simulink model "PolePlacement_Complete_2019"  (R2019a)
settings: Solver=VariableStepAuto  StartTime=0.0  StopTime=10.0  RelTol=1e-3
values from neighbouring files (symbols this model uses):
  k = place(A, B, new_pole)    [PolePlacement_Controller_script.m]
  K_eta = K_en(5)    [PolePlacement_Controller_script.m]
  K_x = K_en(1:4)    [PolePlacement_Controller_script.m]
  Kr = 1/Kdc(1)    [PolePlacement_Controller_script.m]
  L = C_comp*TF(1)    [LQR_Controller.m]    (also in PolePlacement_Controller_script.m = place(sysestc.A',sysestc.C', 10*new_pole)')
  sysestc = d2c(sysest)    [Controller.m]    (also in LQR_Controller.m; PolePlacement_Controller_script.m)
undefined symbols (not defined in the file or in its folder): sigbuilder_block, v_a_max
libraries: simulink_extras x2
settings Model: Creator=jesuc  LastModifiedBy=arco
settings DebuggingCC: SFMachineParentedDataDiag=error

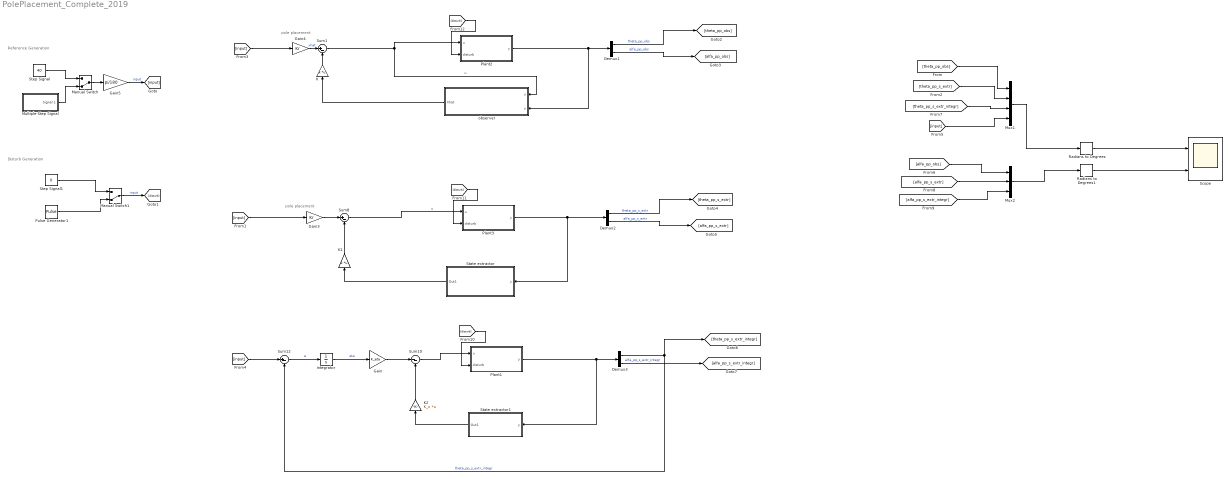
== system PolePlacement_Complete_2019 ==
  note: pole placement
  note: Reference Generation
  note: Disturb Generation
  note: pole placement
  Demux1 : Demux  Outputs=2
  Demux2 : Demux  Outputs=2
  Demux3 : Demux  Outputs=2
  Gain : Gain  Gain=K_eta
  Gain3 : Gain  Gain=Kr
  Gain4 : Gain  Gain=Kr
  Gain5 : Gain  Gain=pi/180
  Integrator : Integrator
  K : Gain  Gain=k  Multiplication=Matrix(K*u)
  K1 : Gain  Gain=k  Multiplication=Matrix(K*u)
  K2 : Gain  Gain=K_x  Multiplication=Matrix(K*u)
  Manual Switch : ManualSwitch  CurrentSetting=0
  Manual Switch1 : ManualSwitch  CurrentSetting=0
  Multiple-Step Signal : Subsystem  Tag=STV Subsys  LoadFcn=sigbuilder_block('load');  StartFcn=sigbuilder_block('start');  StopFcn=sigbuilder_block('stop');  ClipboardFcn=sigbuilder_block('clipboard');  mask(Sigbuilder block){tuvar=[0:10]}
      mask help: Simulink:masks:SigbuilderBlock_MD
      mask init:
      | if ~strcmp(get_param(bdroot(gcbh),'SimulationStatus'),'stopped') tuvar = sigbuilder_block('maskInit'); end
      settings: CopyFcn=sigbuilder_block('copy');  DeleteFcn=sigbuilder_block('delete');  ModelCloseFcn=sigbuilder_block('modelClose');  PreSaveFcn=sigbuilder_block('preSave');  PauseFcn=sigbuilder_block('pause');  ContinueFcn=sigbuilder_block('continue');  NameChangeFcn=sigbuilder_block('namechange');  OpenFcn=sigbuilder_block('open',[437.6 199.2 550.4 400 ]);  CloseFcn=sigbuilder_block('close');
      mask Display: plot(0, 0, 100, 100,[2, 2, 32, 32, 2], [68, 8, 8, 68, 68],[32, 2], [38, 38], [32, 19, 2],[53, 60, 44], [32, 17, 17, 2],[16, 16, 31, 31]);txt = getActiveGroup(gcbh);text(2, 100, txt,'verticalAlignment', 'top');
  Mux1 : Mux
  Mux2 : Mux  Inputs=3
  Plant1 : Subsystem
  Plant2 : Subsystem
  Plant3 : Subsystem
  Pulse Generator1 : DiscretePulseGenerator  PulseType=Time based  Amplitude=.2  Period=1.5  PulseWidth=5
  Radians to Degrees : simulink_extras/Transformations/Radians to Degrees
  Radians to Degrees1 : simulink_extras/Transformations/Radians to Degrees
  Scope : Scope  NumInputPorts=2
  State extractor : Subsystem
  State extractor1 : Subsystem
  Step Signal : Constant  Value=40
  Step Signal1 : Constant  Value=0
  Sum1 : Sum  Inputs=|+-
  Sum10 : Sum  Inputs=|--
  Sum12 : Sum  Inputs=|+-
  Sum8 : Sum  Inputs=|+-
  observer : Subsystem
  wires:
  K/1 -> Sum1/2
  Demux1/1 -> [theta_pp_obs]  "theta_pp_obs"
  Demux1/2 -> [alfa_pp_obs]  "alfa_pp_obs"
  K1/1 -> Sum8/2
  Gain3/1 -> Sum8/1
  Gain4/1 -> Sum1/1  "xhat"
  Mux1/1 -> Radians to Degrees/1
  Multiple-Step Signal/1(Signal 1) -> Manual Switch/2
  Step Signal/1 -> Manual Switch/1
  Manual Switch/1 -> Gain5/1
  Mux2/1 -> Radians to Degrees1/1
  Sum1/1 -> Plant2/1(u), observer/1(u)  "u"
  Step Signal1/1 -> Manual Switch1/1
  Sum10/1 -> Plant1/1(u)
  Integrator/1 -> Gain/1  "eta"
  Sum12/1 -> Integrator/1  "e"
  Demux3/1 -> [theta_pp_s_extr_integr], Sum12/2  "theta_pp_s_extr_integr"
  K2/1 -> Sum10/2
  Gain/1 -> Sum10/1
  State extractor1/1(Out1) -> K2/1
  State extractor/1(Out1) -> K1/1
  Pulse Generator1/1 -> Manual Switch1/2
  Radians to Degrees/1 -> Scope/1
  Radians to Degrees1/1 -> Scope/2
  Gain5/1 -> [input]  "input"
  Manual Switch1/1 -> [disturb]  "input"
  Sum8/1 -> Plant3/1(u)  "u"
  [input] -> Gain4/1
  [input] -> Gain3/1
  [input] -> Sum12/1
  [input] -> Mux1/4
  Plant1/1(y) -> Demux3/1, State extractor1/1(y)
  Plant2/1(y) -> Demux1/1, observer/2(y)
  observer/1(Xhat) -> K/1
  Demux2/2 -> [alfa_pp_s_extr]  "alfa_pp_s_extr"
  Demux2/1 -> [theta_pp_s_extr]  "theta_pp_s_extr"
  Demux3/2 -> [alfa_pp_s_extr_integr]  "alfa_pp_s_extr_integr"
  [theta_pp_obs] -> Mux1/1
  [theta_pp_s_extr] -> Mux1/2
  [theta_pp_s_extr_integr] -> Mux1/3
  [alfa_pp_obs] -> Mux2/1
  [alfa_pp_s_extr] -> Mux2/2
  [alfa_pp_s_extr_integr] -> Mux2/3
  [disturb] -> Plant1/2(disturb)
  [disturb] -> Plant3/2(disturb)
  Plant3/1(y) -> State extractor/1(y), Demux2/1
  [disturb] -> Plant2/2(disturb)

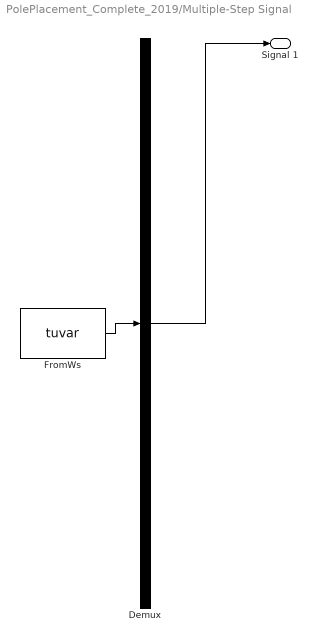
== system PolePlacement_Complete_2019/Multiple-Step Signal ==
  Demux : Demux  Tag=STV Demux  Outputs=1
      settings: DisplayOption=none
  FromWs : FromWorkspace  Tag=STV FromWs  VariableName=tuvar
      SigBuilderData=|
      | common.afterFinalStr = 'Extrapolate'
      | common.sampleTime = 0
      | dataSet.timeRange = [0 10]
      | dataSet.name = 'Group 1'
      | sbobj.Groups.Name = 'Group 1'
      | sbobj.Groups.Signals.Name = 'Signal 1'
      | sbobj.Groups.Signals.XData = [0 1 1 3 3 5 5 7 7 8.5 8.5 10]
      | sbobj.Groups.Signals.YData = [0.005 0.005 40 40 15 15 -30 -30 0 0 23 23]
  Signal 1 : Outport  Tag=STV Outport
  wires:
  Demux/1 -> Signal 1/1
  FromWs/1 -> Demux/1

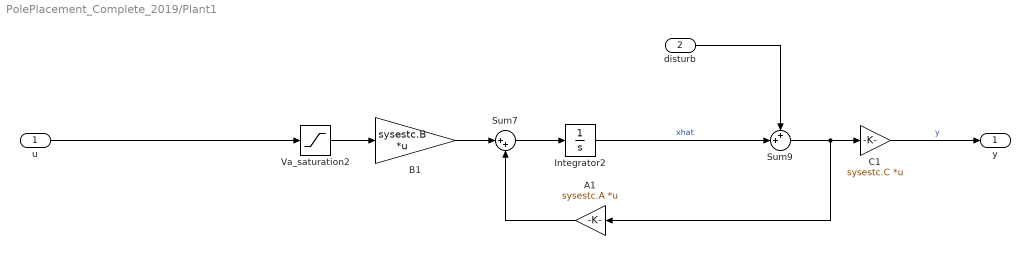
== system PolePlacement_Complete_2019/Plant1 ==
  u : Inport
  disturb : Inport  Port=2
  A1 : Gain  Gain=sysestc.A  Multiplication=Matrix(K*u)
  B1 : Gain  Gain=sysestc.B  Multiplication=Matrix(K*u)
  C1 : Gain  Gain=sysestc.C  Multiplication=Matrix(K*u)
  Integrator2 : Integrator
  Sum7 : Sum  Inputs=|++
  Sum9 : Sum  Inputs=++|
  Va_saturation2 : Saturate  UpperLimit=v_a_max  LowerLimit=-v_a_max
  y : Outport
  wires:
  Sum7/1 -> Integrator2/1
  disturb/1 -> Sum9/1
  B1/1 -> Sum7/1
  Integrator2/1 -> Sum9/2  "xhat"
  C1/1 -> y/1  "y"
  u/1 -> Va_saturation2/1
  A1/1 -> Sum7/2
  Sum9/1 -> A1/1, C1/1
  Va_saturation2/1 -> B1/1

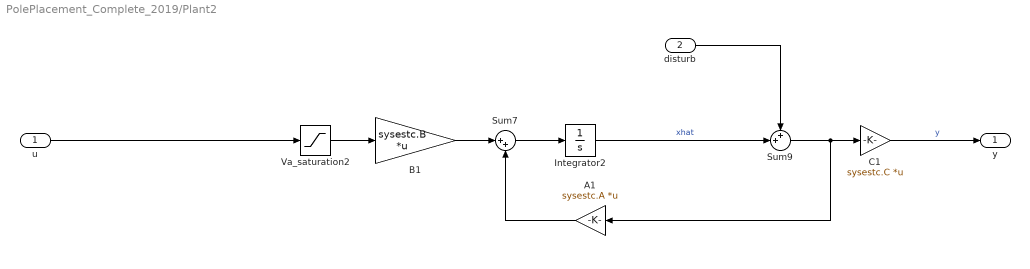
== system PolePlacement_Complete_2019/Plant2 ==
  u : Inport
  disturb : Inport  Port=2
  A1 : Gain  Gain=sysestc.A  Multiplication=Matrix(K*u)
  B1 : Gain  Gain=sysestc.B  Multiplication=Matrix(K*u)
  C1 : Gain  Gain=sysestc.C  Multiplication=Matrix(K*u)
  Integrator2 : Integrator
  Sum7 : Sum  Inputs=|++
  Sum9 : Sum  Inputs=++|
  Va_saturation2 : Saturate  UpperLimit=v_a_max  LowerLimit=-v_a_max
  y : Outport
  wires:
  Sum7/1 -> Integrator2/1
  disturb/1 -> Sum9/1
  B1/1 -> Sum7/1
  Integrator2/1 -> Sum9/2  "xhat"
  C1/1 -> y/1  "y"
  u/1 -> Va_saturation2/1
  A1/1 -> Sum7/2
  Sum9/1 -> A1/1, C1/1
  Va_saturation2/1 -> B1/1

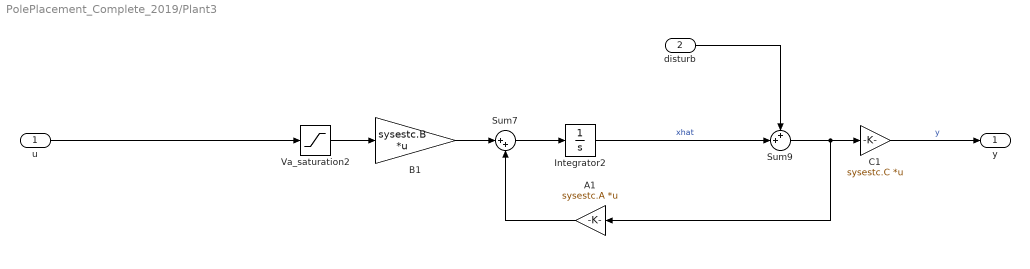
== system PolePlacement_Complete_2019/Plant3 ==
  u : Inport
  disturb : Inport  Port=2
  A1 : Gain  Gain=sysestc.A  Multiplication=Matrix(K*u)
  B1 : Gain  Gain=sysestc.B  Multiplication=Matrix(K*u)
  C1 : Gain  Gain=sysestc.C  Multiplication=Matrix(K*u)
  Integrator2 : Integrator
  Sum7 : Sum  Inputs=|++
  Sum9 : Sum  Inputs=++|
  Va_saturation2 : Saturate  UpperLimit=v_a_max  LowerLimit=-v_a_max
  y : Outport
  wires:
  Sum7/1 -> Integrator2/1
  disturb/1 -> Sum9/1
  B1/1 -> Sum7/1
  Integrator2/1 -> Sum9/2  "xhat"
  C1/1 -> y/1  "y"
  u/1 -> Va_saturation2/1
  A1/1 -> Sum7/2
  Sum9/1 -> A1/1, C1/1
  Va_saturation2/1 -> B1/1

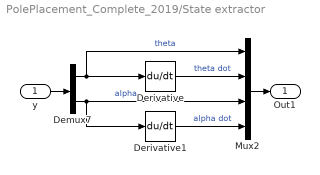
== system PolePlacement_Complete_2019/State extractor ==
  y : Inport
  Demux7 : Demux  Outputs=2
  Derivative : Derivative
  Derivative1 : Derivative
  Mux2 : Mux
  Out1 : Outport
  wires:
  y/1 -> Demux7/1
  Derivative1/1 -> Mux2/4  "alpha dot"
  Derivative/1 -> Mux2/2  "theta dot"
  Demux7/1 -> Mux2/1, Derivative/1  "theta"
  Demux7/2 -> Derivative1/1, Mux2/3  "alpha"
  Mux2/1 -> Out1/1

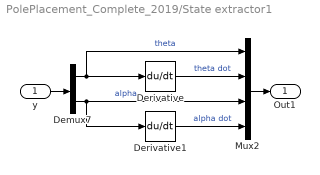
== system PolePlacement_Complete_2019/State extractor1 ==
  y : Inport
  Demux7 : Demux  Outputs=2
  Derivative : Derivative
  Derivative1 : Derivative
  Mux2 : Mux
  Out1 : Outport
  wires:
  y/1 -> Demux7/1
  Derivative1/1 -> Mux2/4  "alpha dot"
  Derivative/1 -> Mux2/2  "theta dot"
  Demux7/1 -> Mux2/1, Derivative/1  "theta"
  Demux7/2 -> Derivative1/1, Mux2/3  "alpha"
  Mux2/1 -> Out1/1

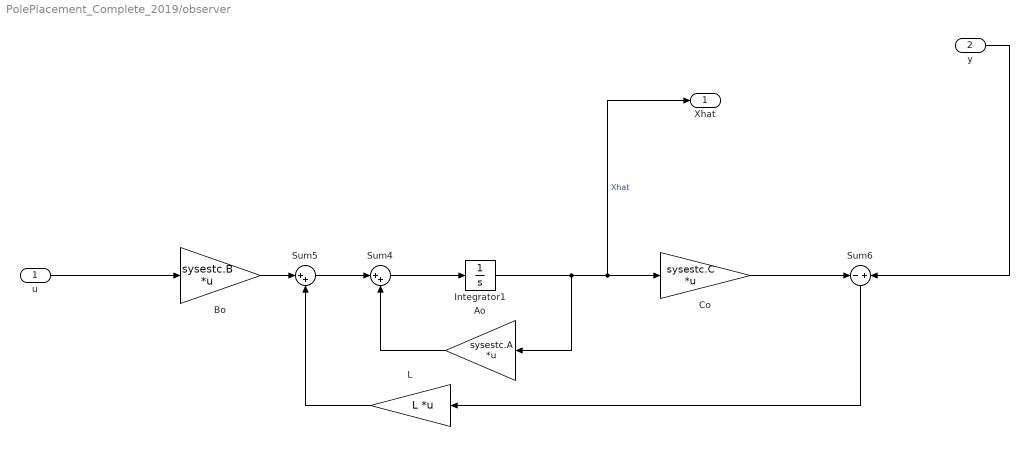
== system PolePlacement_Complete_2019/observer ==
  u : Inport
  y : Inport  Port=2
  Ao : Gain  Gain=sysestc.A  Multiplication=Matrix(K*u)
  Bo : Gain  Gain=sysestc.B  Multiplication=Matrix(K*u)
  Co : Gain  Gain=sysestc.C  Multiplication=Matrix(K*u)
  Integrator1 : Integrator
  L : Gain  Gain=L  Multiplication=Matrix(K*u)
  Sum4 : Sum  Inputs=|++
  Sum5 : Sum  Inputs=|++
  Sum6 : Sum  Inputs=-+
  Xhat : Outport
  wires:
  y/1 -> Sum6/2
  Ao/1 -> Sum4/2
  Sum4/1 -> Integrator1/1
  u/1 -> Bo/1
  Co/1 -> Sum6/1
  Sum6/1 -> L/1
  Bo/1 -> Sum5/1
  L/1 -> Sum5/2
  Integrator1/1 -> Xhat/1, Co/1, Ao/1  "Xhat"
  Sum5/1 -> Sum4/1
